simulink library "pd_control_lib"  (R2016b)
settings: Solver=ode45  StartTime=0.0  StopTime=10.0  RelTol=1e-3  EnableMultiTasking=on
libraries: aerolibutil x2
settings Model: Creator=Taylor  LastModifiedBy=taylorreynolds
settings DataIOCC: LimitDataPoints=on
settings OptimizationCC: LifeSpan=inf
settings DebuggingCC: AllowSymbolicDim=off  SFUnexpectedBacktrackingDiag=warning  SFNoUnconditionalDefaultTransitionDiag=warning  SFExecutionAtInitializationDiag=none
settings GRTTargetCC: TargetLangStandard=C89/C90 (ANSI)  GeneratePreprocessorConditionals=Disable all
settings ConfigComp: CovMetricSettings=dw  CovHtmlReporting=on  CovSaveCumulativeToWorkspaceVar=on  CovSaveSingleToWorkspaceVar=on  CovExternalEMLEnable=off

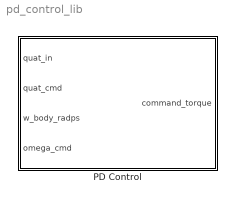
== system pd_control_lib ==
  PD Control : Subsystem

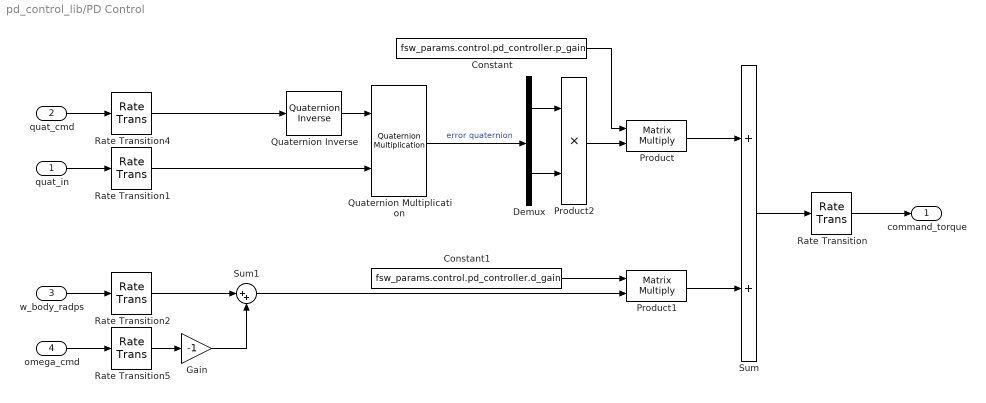
== system pd_control_lib/PD Control ==
  quat_in : Inport
  quat_cmd : Inport  Port=2
  w_body_radps : Inport  Port=3
  omega_cmd : Inport  Port=4
  Constant : Constant  Value=fsw_params.control.pd_controller.p_gain
  Constant1 : Constant  Value=fsw_params.control.pd_controller.d_gain
  Demux : Demux  Outputs=[1 3]
  Gain : Gain  Gain=-1
  Product : Product  Multiplication=Matrix(*)
  Product1 : Product  Multiplication=Matrix(*)
  Product2 : Product
  Quaternion Inverse : aerolibutil/Quaternion Inverse
  Quaternion Multiplication : aerolibutil/Quaternion Multiplication
  Rate Transition : RateTransition  X0=fsw_params.control.pd_controller.ic.rt_command_torque
  Rate Transition1 : RateTransition  X0=fsw_params.control.pd_controller.ic.rt_quat_in  OutPortSampleTime=fsw_params.control.pd_controller.sample_time_s
  Rate Transition2 : RateTransition  X0=fsw_params.control.pd_controller.ic.rt_w_body_radps  OutPortSampleTime=fsw_params.control.pd_controller.sample_time_s
  Rate Transition4 : RateTransition  X0=fsw_params.control.pd_controller.ic.rt_quat_in  OutPortSampleTime=fsw_params.control.pd_controller.sample_time_s
  Rate Transition5 : RateTransition  X0=fsw_params.control.pd_controller.ic.rt_w_body_radps  OutPortSampleTime=fsw_params.control.pd_controller.sample_time_s
  Sum : Sum
  Sum1 : Sum  Inputs=|++
  command_torque : Outport
  wires:
  Constant1/1 -> Product1/1
  Constant/1 -> Product/1
  quat_cmd/1 -> Rate Transition4/1
  Quaternion Inverse/1 -> Quaternion Multiplication/1
  quat_in/1 -> Rate Transition1/1
  Quaternion Multiplication/1 -> Demux/1  "error quaternion"
  Demux/1 -> Product2/1
  w_body_radps/1 -> Rate Transition2/1
  Demux/2 -> Product2/2
  Product/1 -> Sum/1
  Product1/1 -> Sum/2
  Sum/1 -> Rate Transition/1
  Rate Transition/1 -> command_torque/1
  Rate Transition1/1 -> Quaternion Multiplication/2
  Rate Transition4/1 -> Quaternion Inverse/1
  omega_cmd/1 -> Rate Transition5/1
  Rate Transition2/1 -> Sum1/1
  Rate Transition5/1 -> Gain/1
  Gain/1 -> Sum1/2
  Sum1/1 -> Product1/2
  Product2/1 -> Product/2
